simulink model "M003_refor_meca"  (R2021a)
settings: Solver=VariableStepAuto  StartTime=0.0  StopTime=100  RelTol=1e-3
undefined symbols (not defined in the file or in its folder): params
settings Model: Creator=djoroya  LastModifiedBy=djoroya

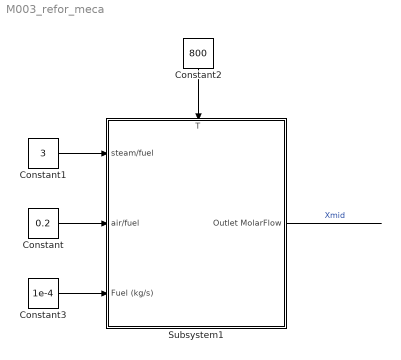
== system M003_refor_meca ==
  Constant : Constant  Value=0.2
  Constant1 : Constant  Value=3
  Constant2 : Constant  Value=800
  Constant3 : Constant  Value=1e-4
  Subsystem1 : Subsystem
      settings: PortSchema="{\"entries\":[{\"content\":{\"sides\":[{\"content\":{\"connectorIds\":[\"In1\",\"In2\",\"In3\"]},\"type\":\"ConnectorPlacement.EquallySpacedRectSide\",\"uuid\":\"bba98e9a-4a8f-433d-80b6-6443373beb37\"},{\"content\":{\"connectorIds\":[\"Out1\"],\"side\":\"RIGHT\"},\"type\":\"ConnectorPlacement.EquallySpacedRectSide\",\"uuid\":\"bb8208fa-3ad6-4550-bb87-9c458da504c5\"},{\"content\":{\"connectorIds\":[\"In4\"],\"side\":\"TOP\"},\"type\":\"ConnectorPlacement.EquallySpacedRectSide\",\"uuid\":\"10760c79-2681-4834-b090-bc5e1ffe83d8\"}]},\"type\":\"ConnectorPlacement.EquallySpacedConnector\",\"uuid\":\"c7bbf7d3-64d5-4f0e-88ff-bb50ba74e7ab\"}],\"packageUris\":[\"http://schema.mathworks.com/mf0/Connector/R2020b\"],\"version\":\"1.0\"}"
  wires:
  Subsystem1/1(Outlet MolarFlow) -> ?  "Xmid"
  Constant/1 -> Subsystem1/2(air/fuel)
  Constant3/1 -> Subsystem1/3(Fuel (kg/s))
  Constant1/1 -> Subsystem1/1(steam/fuel)
  Constant2/1 -> Subsystem1/4(T)

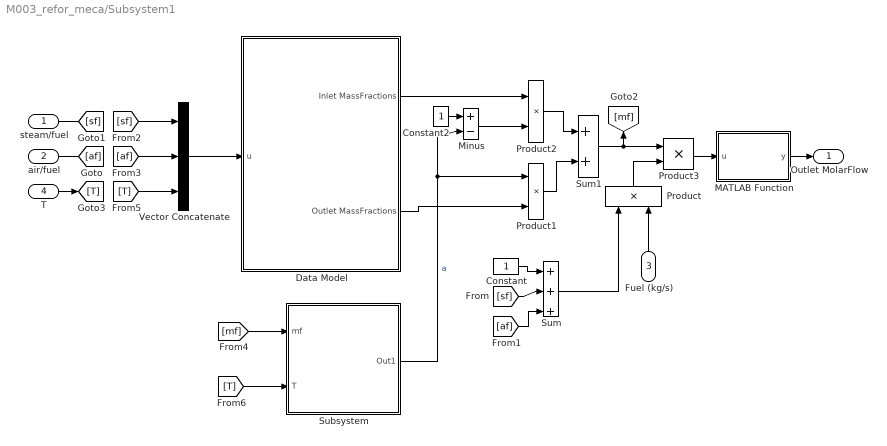
== system M003_refor_meca/Subsystem1 ==
  steam/fuel : Inport
  air/fuel : Inport  Port=2
  Fuel (kg/s) : Inport  Port=3
  T : Inport  Port=4
  Constant : Constant
  Constant2 : Constant
  Data Model : Subsystem
  MATLAB Function : MATLAB Function  TreatAsAtomicUnit=on
  Minus : Sum  Inputs=+-
  Product{,1..3} (4 alike) : Product
  Subsystem : Subsystem
  Sum : Sum  Inputs=|+++
  Sum1 : Sum  Inputs=|++
  Vector Concatenate : Concatenate  NumInputs=3
  Outlet MolarFlow : Outport
  wires:
  Constant2/1 -> Minus/1
  Product1/1 -> Sum1/2
  Minus/1 -> Product2/2
  [af] -> Vector Concatenate/2
  [sf] -> Vector Concatenate/1
  Product2/1 -> Sum1/1
  [sf] -> Sum/2
  steam/fuel/1 -> [sf]
  Product/1 -> Product3/2
  air/fuel/1 -> [af]
  Sum1/1 -> Product3/1, [mf]
  [af] -> Sum/3
  Constant/1 -> Sum/1
  Vector Concatenate/1 -> Data Model/1(u)
  Data Model/1(Inlet MassFractions) -> Product2/1
  Data Model/2(Outlet MassFractions) -> Product1/2
  Fuel (kg/s)/1 -> Product/2
  Sum/1 -> Product/1
  T/1 -> [T]
  [T] -> Vector Concatenate/3
  Subsystem/1(Out1) -> Minus/2, Product1/1  "a"
  [mf] -> Subsystem/1(mf)
  [T] -> Subsystem/2(T)
  Product3/1 -> MATLAB Function/1(u)
  MATLAB Function/1(y) -> Outlet MolarFlow/1

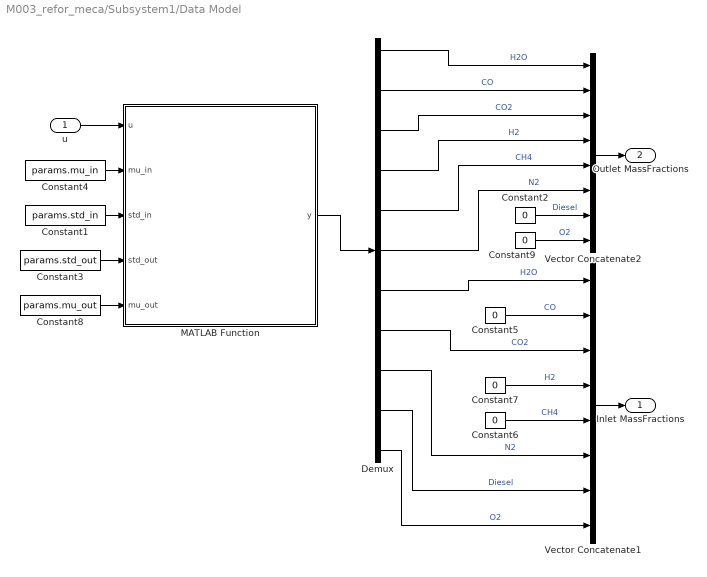
== system M003_refor_meca/Subsystem1/Data Model ==
  u : Inport
  Constant1 : Constant  Value=params.std_in
  Constant{2,5..7,9} (5 alike) : Constant  Value=0
  Constant3 : Constant  Value=params.std_out
  Constant4 : Constant  Value=params.mu_in
  Constant8 : Constant  Value=params.mu_out
  Demux : Demux  Outputs=11
  MATLAB Function : MATLAB Function  TreatAsAtomicUnit=on
  Vector Concatenate1 : Concatenate  NumInputs=8
  Vector Concatenate2 : Concatenate  NumInputs=8
  Inlet MassFractions : Outport
  Outlet MassFractions : Outport  Port=2
  wires:
  Vector Concatenate1/1 -> Inlet MassFractions/1
  Constant6/1 -> Vector Concatenate1/5  "CH4"
  Demux/4 -> Vector Concatenate2/4  "H2"
  Demux/1 -> Vector Concatenate2/1  "H2O"
  Demux/2 -> Vector Concatenate2/2  "CO"
  Vector Concatenate2/1 -> Outlet MassFractions/1
  Constant5/1 -> Vector Concatenate1/2  "CO"
  Demux/5 -> Vector Concatenate2/5  "CH4"
  Constant4/1 -> MATLAB Function/2(mu_in)
  u/1 -> MATLAB Function/1(u)
  Constant1/1 -> MATLAB Function/3(std_in)
  Constant3/1 -> MATLAB Function/4(std_out)
  Constant8/1 -> MATLAB Function/5(mu_out)
  Demux/3 -> Vector Concatenate2/3  "CO2"
  MATLAB Function/1(y) -> Demux/1
  Demux/6 -> Vector Concatenate2/6  "N2"
  Demux/7 -> Vector Concatenate1/1  "H2O"
  Constant2/1 -> Vector Concatenate2/7  "Diesel"
  Demux/8 -> Vector Concatenate1/3  "CO2"
  Demux/9 -> Vector Concatenate1/6  "N2"
  Demux/10 -> Vector Concatenate1/7  "Diesel"
  Constant7/1 -> Vector Concatenate1/4  "H2"
  Demux/11 -> Vector Concatenate1/8  "O2"
  Constant9/1 -> Vector Concatenate2/8  "O2"

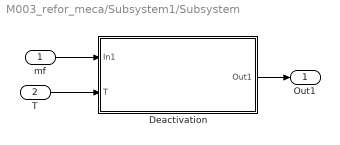
== system M003_refor_meca/Subsystem1/Subsystem ==
  mf : Inport
  T : Inport  Port=2
  Deactivation : Subsystem  mask{k0=0.024, k=[0 0 0 0 0 0 0 ]', nd=1, Kw_ast=0, Ew=0}
  Out1 : Outport
  wires:
  T/1 -> Deactivation/2(T)
  mf/1 -> Deactivation/1(In1)
  Deactivation/1(Out1) -> Out1/1

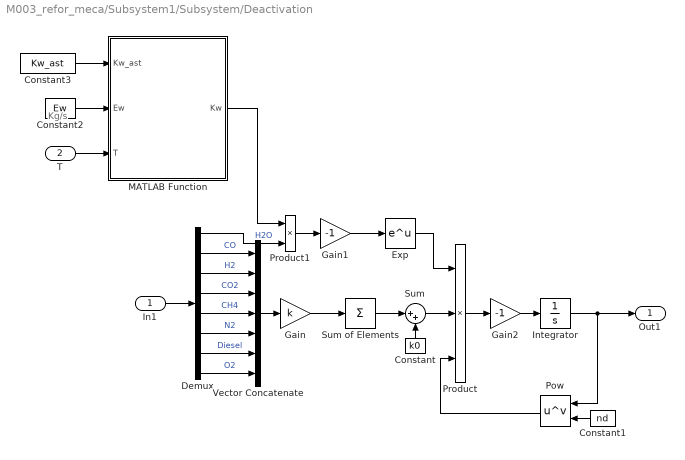
== system M003_refor_meca/Subsystem1/Subsystem/Deactivation ==
  note: Kg/s
  In1 : Inport
  T : Inport  Port=2
  Constant : Constant  Value=k0
  Constant1 : Constant  Value=nd
  Constant2 : Constant  Value=Ew
  Constant3 : Constant  Value=Kw_ast
  Demux : Demux  Outputs=8
  Exp : Math  SaturateOnIntegerOverflow=on
  Gain : Gain  Gain=k
  Gain1 : Gain  Gain=-1
  Gain2 : Gain  Gain=-1
  Integrator : Integrator  InitialCondition=1
  MATLAB Function : MATLAB Function  TreatAsAtomicUnit=on
  Pow : Math  Operator=pow  RndMeth=Zero  SaturateOnIntegerOverflow=on
  Product : Product  Inputs=3
  Product1 : Product
  Sum : Sum  Inputs=|++
  Sum of Elements : Sum  Inputs=+
  Vector Concatenate : Concatenate  NumInputs=7
  Out1 : Outport
  wires:
  Integrator/1 -> Out1/1, Pow/1
  In1/1 -> Demux/1
  Demux/6 -> Vector Concatenate/5  "N2"
  Demux/5 -> Vector Concatenate/4  "CH4"
  Demux/4 -> Vector Concatenate/3  "CO2"
  Demux/3 -> Vector Concatenate/2  "H2"
  Demux/2 -> Vector Concatenate/1  "CO"
  Vector Concatenate/1 -> Gain/1
  Constant/1 -> Sum/2
  Sum/1 -> Product/2
  Demux/1 -> Product1/2  "H2O"
  Exp/1 -> Product/1
  Pow/1 -> Product/3
  Constant1/1 -> Pow/2
  Gain/1 -> Sum of Elements/1
  Sum of Elements/1 -> Sum/1
  Product/1 -> Gain2/1
  Gain2/1 -> Integrator/1
  Demux/7 -> Vector Concatenate/6  "Diesel"
  T/1 -> MATLAB Function/3(T)
  Constant2/1 -> MATLAB Function/2(Ew)
  Constant3/1 -> MATLAB Function/1(Kw_ast)
  MATLAB Function/1(Kw) -> Product1/1
  Product1/1 -> Gain1/1
  Gain1/1 -> Exp/1
  Demux/8 -> Vector Concatenate/7  "O2"

== matlab function M003_refor_meca/Subsystem1/MATLAB Function ==
  data: u input; y output
function y = fcn(u)


p.H2  = 2e-3;  % kg/mol
p.O2  = 32e-3; % kg/mol
p.H2O = 18e-3; % kg/mol
p.N2  = 28e-3; % kg/mol
p.CO  = 28e-3; % kg/mol
p.CH4 = 16e-3; % kg/mol
p.CO2 = 44e-3; % kg/mol
%p.Air = 28.9647-3;	 % kg/mol;
p.Diesel = 142e-3;	 % kg/mol;

H2O = u(1)/p.H2O;
CO  = u(2)/p.CO;
CO2 = u(3)/p.CO2;
H2  = u(4)/p.H2;
CH4 = u(5)/p.CH4;
N2 = u(6)/p.N2;
Diesel = u(7)/p.Diesel;
O2 = u(8)/p.O2;

y = [H2 O2 H2O N2 CO CH4 CO2 Diesel]';

== matlab function M003_refor_meca/Subsystem1/Data Model/MATLAB Function ==
  data: u input; y output; mu_in input; std_in input; std_out input; mu_out input
function y = fcn(u,mu_in,std_in,std_out,mu_out)

y = REFORMER_mf((u - mu_in)./std_in).*std_out + mu_out;

== matlab function M003_refor_meca/Subsystem1/Subsystem/Deactivation/MATLAB Function ==
  data: Kw_ast input; Kw output; Ew input; T input
function Kw = fcn(Kw_ast,Ew,T)

R = 8.314472;% J/(mol K) 

Kw = Kw_ast*exp(-Ew/R*(1/(T+273.15) - 1/573));
